simulink library "pilotlib"  (Simulink 3.00)
settings Model: Creator=sven  LastModifiedBy=sven

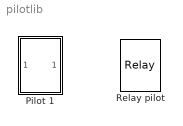
== system pilotlib ==
  Pilot 1 : Subsystem
  Relay pilot : Relay  OnSwitchValue=eps  OffSwitchValue=-eps  OnOutputValue=0.2  OffOutputValue=-0.2

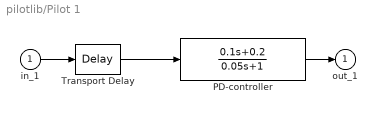
== system pilotlib/Pilot 1 ==
  in_1 : Inport  Port=1  PortWidth=-1  SampleTime=-1  DataType=auto
      settings: SignalType=auto
  PD-controller : TransferFcn  Numerator=[0.1 0.2]  Denominator=[0.05 1]
  Transport Delay : TransportDelay  DelayTime=0.3  InitialInput=0  BufferSize=1024
  out_1 : Outport  Port=1  InitialOutput=0
  wires:
  PD-controller/1 -> out_1/1
  Transport Delay/1 -> PD-controller/1
  in_1/1 -> Transport Delay/1
